simulink library "INT_CrCLmp_DD"  (R2016b)
settings: Solver=VariableStepAuto  StartTime=0.0  StopTime=10.0  RelTol=1e-3
settings Model: Creator=xinchangran  LastModifiedBy=xinchangran

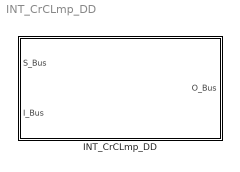
== system INT_CrCLmp_DD ==
  INT_CrCLmp_DD : Subsystem

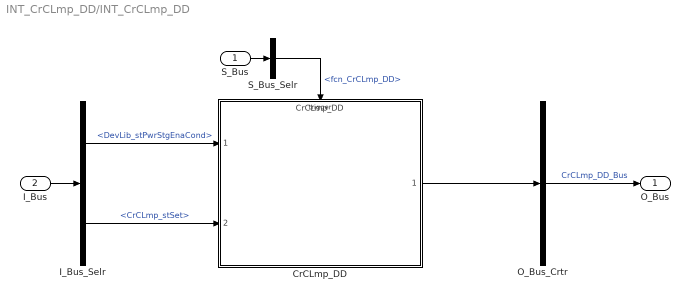
== system INT_CrCLmp_DD/INT_CrCLmp_DD ==
  S_Bus : Inport
  I_Bus : Inport  Port=2
  CrCLmp_DD : ModelReference  ModelNameDialog=CrCLmp_DD  SimulationMode=Normal  ModelReferenceVersion=1.9  TriggerPortName=function  TriggerPortTriggerType=function-call  TriggerPortStatesWhenEnabling=held
  I_Bus_Selr : BusSelector  OutputSignals=DevLib_stPwrStgEnaCond,CrCLmp_stSet
  O_Bus_Crtr : BusCreator  Inputs=1
  S_Bus_Selr : BusSelector  OutputSignals=fcn_CrCLmp_DD
  O_Bus : Outport
  wires:
  S_Bus_Selr/1 -> CrCLmp_DD/Trigger  "<fcn_CrCLmp_DD>"
  S_Bus/1 -> S_Bus_Selr/1
  I_Bus/1 -> I_Bus_Selr/1
  I_Bus_Selr/1 -> CrCLmp_DD/1  "<DevLib_stPwrStgEnaCond>"
  I_Bus_Selr/2 -> CrCLmp_DD/2  "<CrCLmp_stSet>"
  O_Bus_Crtr/1 -> O_Bus/1  "CrCLmp_DD_Bus"
  CrCLmp_DD/1 -> O_Bus_Crtr/1
